simulink subsystem "Nom_AeroProp"  (R2024b)
settings: Solver=VariableStepAuto  StartTime=0.0  StopTime=10.0  RelTol=1e-3
undefined symbols (not defined in the file or in its folder): SimIn, SimPar
libraries: starslibAxisTransformations x1
settings Model: Creator=macheson  LastModifiedBy=macheson

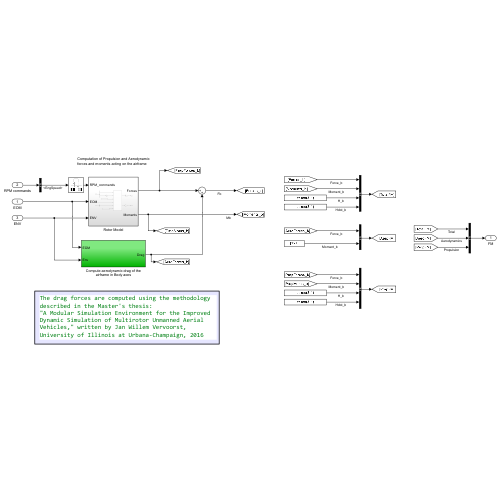
[thumbnail: Simulink's stored preview of the top-level diagram]
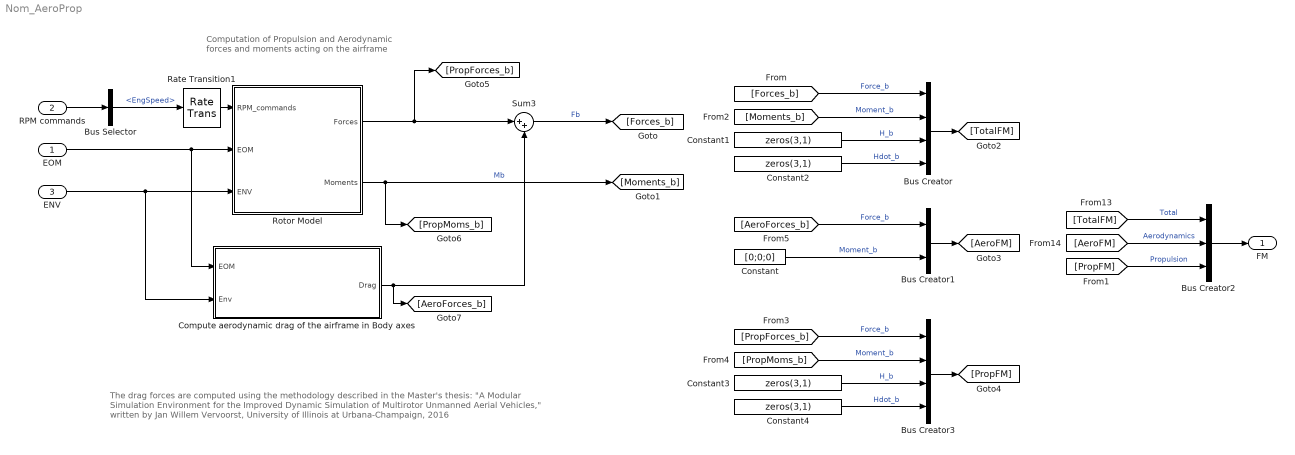
== system Nom_AeroProp ==
  note: The drag forces are computed using the methodology described in the Master's thesis:
      | "A Modular Simulation Environment for the Improved Dynamic Simulation of Multirotor Unmanned Aerial Vehicles," written by Jan Willem Vervoorst,
      | University of Illinois at Urbana-Champaign, 2016
  note: Computation of Propulsion and Aerodynamic
      | forces and moments acting on the airframe
  EOM : Inport
  RPM commands : Inport  Port=2
  ENV : Inport  Port=3
  Bus Creator : BusCreator  Inputs=4
  Bus Creator1 : BusCreator  Inputs=2
  Bus Creator2 : BusCreator  Inputs=3  OutDataTypeStr=Bus: BUS_FORCE_MOMENT
  Bus Creator3 : BusCreator  Inputs=4
  Bus Selector : BusSelector  OutputSignals=EngSpeed
  Compute aerodynamic drag of the airframe in Body axes : Subsystem
  Constant : Constant  Value=[0;0;0]  VectorParams1D=off
  Constant{1..4} (4 alike) : Constant  Value=zeros(3,1)  VectorParams1D=off
  Rate Transition1 : RateTransition  InitialCondition=SimIn.IC.rpm_init  OutPortSampleTime=SimIn.model_params.sim_rate
  Rotor Model : Subsystem
  Sum3 : Sum  Inputs=|++
  FM : Outport  VectorParamsAs1DForOutWhenUnconnected=off
  wires:
  Compute aerodynamic drag of the airframe in Body axes/1(Drag) -> Sum3/2, [AeroForces_b]
  ENV/1 -> Compute aerodynamic drag of the airframe in Body axes/2(Env), Rotor Model/3(ENV)
  [TotalFM] -> Bus Creator2/1  "Total"
  [AeroForces_b] -> Bus Creator1/1  "Force_b"
  Constant4/1 -> Bus Creator3/4  "Hdot_b"
  [Moments_b] -> Bus Creator/2  "Moment_b"
  Constant1/1 -> Bus Creator/3  "H_b"
  Sum3/1 -> [Forces_b]  "Fb"
  Constant2/1 -> Bus Creator/4  "Hdot_b"
  Bus Creator/1 -> [TotalFM]
  Constant/1 -> Bus Creator1/2  "Moment_b"
  Constant3/1 -> Bus Creator3/3  "H_b"
  [Forces_b] -> Bus Creator/1  "Force_b"
  EOM/1 -> Compute aerodynamic drag of the airframe in Body axes/1(EOM), Rotor Model/2(EOM)
  Rotor Model/2(Moments) -> [Moments_b], [PropMoms_b]  "Mb"
  [AeroFM] -> Bus Creator2/2  "Aerodynamics"
  Bus Creator2/1 -> FM/1
  [PropMoms_b] -> Bus Creator3/2  "Moment_b"
  Bus Creator1/1 -> [AeroFM]
  [PropForces_b] -> Bus Creator3/1  "Force_b"
  Rotor Model/1(Forces) -> [PropForces_b], Sum3/1
  [PropFM] -> Bus Creator2/3  "Propulsion"
  Bus Creator3/1 -> [PropFM]
  RPM commands/1 -> Bus Selector/1
  Bus Selector/1 -> Rate Transition1/1  "<EngSpeed>"
  Rate Transition1/1 -> Rotor Model/1(RPM_commands)

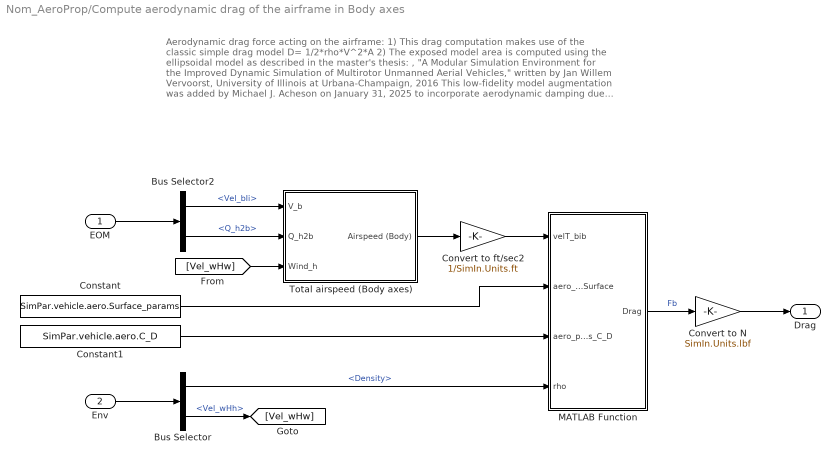
== system Nom_AeroProp/Compute aerodynamic drag of the airframe in Body axes ==
  note: Aerodynamic drag force acting on the airframe:
      | 1) This drag computation makes use of the classic
      | simple drag model D= 1/2*rho*V^2*A
      | 2) The exposed model area is computed using the ellipsoidal
      | model as described in the master's thesis: , "A Modular Simulation Environment for the Improved Dynamic Simulation of Multirotor Unmanned Aerial Vehicles," written by Jan Willem Vervoorst, University of Illinois at Urbana-Champaign, 2016
      |
      | This low-fidelity model augmentation was added by Michael J. Acheson on January 31, 2025 to incorporate aerodynamic damping due to drag into the simple BAM aero-propulsive model.
  EOM : Inport
  Env : Inport  Port=2
  Bus Selector : BusSelector  OutputSignals=Atmosphere.Density,Wind.Vel_wHh
  Bus Selector2 : BusSelector  OutputSignals=InertialData.Vel_bIi,WorldRelativeData.Q_h2b
  Constant : Constant  Value=SimPar.vehicle.aero.Surface_params
  Constant1 : Constant  Value=SimPar.vehicle.aero.C_D
  Convert to N : Gain  Gain=SimIn.Units.lbf
  Convert to ft/sec2 : Gain  Gain=1/SimIn.Units.ft
  MATLAB Function : MATLAB Function  TreatAsAtomicUnit=on
  Total airspeed (Body axes) : Subsystem
  Drag : Outport  VectorParamsAs1DForOutWhenUnconnected=off
  wires:
  MATLAB Function/1(Drag) -> Convert to N/1  "Fb"
  EOM/1 -> Bus Selector2/1
  Constant/1 -> MATLAB Function/2(aero_params_Surface)
  Bus Selector2/1 -> Total airspeed (Body axes)/1(V_b)  "<Vel_bIi>"
  Bus Selector2/2 -> Total airspeed (Body axes)/2(Q_h2b)  "<Q_h2b>"
  [Vel_wHw] -> Total airspeed (Body axes)/3(Wind_h)
  Total airspeed (Body axes)/1(Airspeed (Body)) -> Convert to ft/sec2/1
  Env/1 -> Bus Selector/1
  Bus Selector/1 -> MATLAB Function/4(rho)  "<Density>"
  Constant1/1 -> MATLAB Function/3(aero_params_C_D)
  Bus Selector/2 -> [Vel_wHw]  "<Vel_wHh>"
  Convert to N/1 -> Drag/1
  Convert to ft/sec2/1 -> MATLAB Function/1(velT_bib)

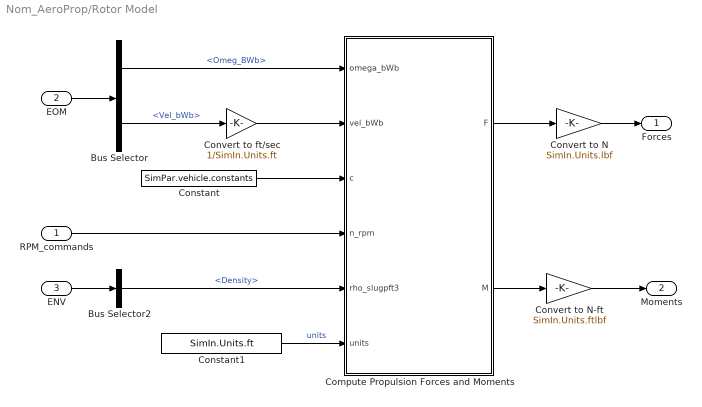
== system Nom_AeroProp/Rotor Model ==
  RPM_commands : Inport
  EOM : Inport  Port=2
  ENV : Inport  Port=3
  Bus Selector : BusSelector  OutputSignals=AirRelativeData.Omeg_BWb,AirRelativeData.Vel_bWb
  Bus Selector2 : BusSelector  OutputSignals=Atmosphere.Density
  Compute Propulsion Forces and Moments : MATLAB Function  TreatAsAtomicUnit=on
  Constant : Constant  Value=SimPar.vehicle.constants  OutDataTypeStr=Bus: BUS_PARAM_constants
  Constant1 : Constant  Value=SimIn.Units.ft
  Convert to N : Gain  Gain=SimIn.Units.lbf
  Convert to N-ft : Gain  Gain=SimIn.Units.ftlbf
  Convert to ft/sec : Gain  Gain=1/SimIn.Units.ft
  Forces : Outport
  Moments : Outport  Port=2
  wires:
  Bus Selector/1 -> Compute Propulsion Forces and Moments/1(omega_bWb)  "<Omeg_BWb>"
  Bus Selector/2 -> Convert to ft/sec/1  "<Vel_bWb>"
  RPM_commands/1 -> Compute Propulsion Forces and Moments/4(n_rpm)
  EOM/1 -> Bus Selector/1
  ENV/1 -> Bus Selector2/1
  Compute Propulsion Forces and Moments/1(F) -> Convert to N/1
  Compute Propulsion Forces and Moments/2(M) -> Convert to N-ft/1
  Bus Selector2/1 -> Compute Propulsion Forces and Moments/5(rho_slugpft3)  "<Density>"
  Constant/1 -> Compute Propulsion Forces and Moments/3(c)
  Constant1/1 -> Compute Propulsion Forces and Moments/6(units)  "units"
  Convert to N/1 -> Forces/1
  Convert to N-ft/1 -> Moments/1
  Convert to ft/sec/1 -> Compute Propulsion Forces and Moments/2(vel_bWb)

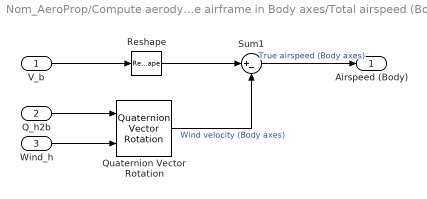
== system Nom_AeroProp/Compute aerodynamic drag of the airframe in Body axes/Total airspeed (Body axes) ==
  V_b : Inport
  Q_h2b : Inport  Port=2
  Wind_h : Inport  Port=3
  Quaternion Vector Rotation : starslibAxisTransformations/Quaternion Vector Rotation  n=0
  Reshape : Reshape  OutputDimensionality=Column vector (2-D)
  Sum1 : Sum  Inputs=|+-
  Airspeed (Body) : Outport  VectorParamsAs1DForOutWhenUnconnected=off
  wires:
  Q_h2b/1 -> Quaternion Vector Rotation/1
  Wind_h/1 -> Quaternion Vector Rotation/2
  Quaternion Vector Rotation/1 -> Sum1/2  "Wind velocity (Body axes)"
  Reshape/1 -> Sum1/1
  V_b/1 -> Reshape/1
  Sum1/1 -> Airspeed (Body)/1  "True airspeed (Body axes)"

== matlab function Nom_AeroProp/Compute aerodynamic drag of the airframe in Body axes/MATLAB Function ==
  data: velT_bib input; aero_params_Surface input; Drag output; aero_params_C_D input; rho input
function Drag  = Quad_Drag(velT_bib, aero_params_Surface, aero_params_C_D, rho)

% function [X_lbf, Y_lbf, Z_lbf] = quad_drag(velT_bib, aero_params, rho)
% This file computes a model of aerodynamic drag. The drag forces are
% computed using the methodology described in the Master's thesis:
% "A Modular Simulation Environment for the Improved Dynamic Simulation
%  of Multirotor Unmanned Aerial Vehicles," written by Jan Willem Vervoorst,
% University of Illinois at Urbana-Champain, 2016
%
% Inputs
%   velT_bib: (TAS) velocity of the multirotor cg wrt inertial frame (non-spinning
%       Earth) expressed in body frame coordinates
%   x: states 
%       = [phi,theta,psi,... %(rad)
%          u,v,w,...         %(ft/s)
%          p,q,r,...         %(rad/s)
%          x,y,z]            %(ft)
%   aero_params: structure of quadrotor surface area and drag parameters
%   rho:     atmosphere density (in units slug/ft3)
%
% Written by Michael J. Acheson, Dynamics and Control Branch (D-316)
% NASA Langley Research Center
%
% History:
% 1/31/2025, MJA Initial Version

% Non-linear (rigid body) states and controls
%   x: states 
%       = [phi,theta,psi,... %(rad)
%          u,v,w,...         %(ft/s)
%          p,q,r,...         %(rad/s)
%          x,y,z]            %(ft)
%   u: control inputs vector (rad/sec)

% Compute "exposed model surface area" using ellipsoidal model
scale_fac = 1/sqrt(sum((velT_bib./aero_params_Surface).^2));
MR_Surf_Area = vecnorm(velT_bib*scale_fac);

if all(velT_bib==0)
    Drag = [0;0;0];
else
    % Compute drag force using simplified model: Drag = 1/2*rho*V^2*Area
    Drag = -velT_bib/vecnorm(velT_bib)*rho*(velT_bib'*velT_bib)*aero_params_C_D*MR_Surf_Area/2;
end
% Map drag to function outputs
% X_lbf = Drag(1);
%Y_lbf = Drag(2);
% Z_lbf = Drag(3);

end

== matlab function Nom_AeroProp/Rotor Model/Compute Propulsion Forces and Moments ==
  data: omega_bWb input; vel_bWb input; c input; n_rpm input; rho_slugpft3 input; F output; M output; units input
function [F, M] = compute_prop(omega_bWb, vel_bWb, c, n_rpm, rho_slugpft3, units)

 [F, M] = compute_multirotor_FM(vel_bWb, omega_bWb, n_rpm, rho_slugpft3, c, units);
